simulink model "full_obs"  (Simulink 7.3)
settings: Solver=ode3  StartTime=0.0  StopTime=1500  FixedStep=1  RelTol=1e-3
settings Model: Creator=alkis  LastModifiedBy=alkis
settings DataIOCC: MaxDataPoints=10000  SaveState=on

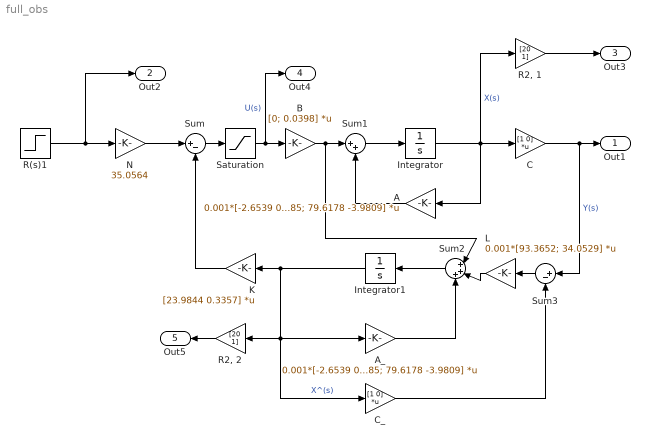
== system full_obs ==
  A : Gain  Gain=0.001*[-2.6539 0.0885; 79.6178 -3.9809]  Multiplication=Matrix(K*u)  ParameterDataType=fixdt(1, 16)  ParameterScaling=2^0  OutDataType=fixdt(1, 16)  OutScaling=2^0
  A_ : Gain  Gain=0.001*[-2.6539 0.0885; 79.6178 -3.9809]  Multiplication=Matrix(K*u)  ParameterDataType=fixdt(1, 16)  ParameterScaling=2^0  OutDataType=fixdt(1, 16)  OutScaling=2^0
  B : Gain  Gain=[0; 0.0398]  Multiplication=Matrix(K*u)  ParameterDataType=fixdt(1, 16)  ParameterScaling=2^0  OutDataType=fixdt(1, 16)  OutScaling=2^0
  C : Gain  Gain=[1 0]  Multiplication=Matrix(K*u)  ParameterDataType=fixdt(1, 16)  ParameterScaling=2^0  OutDataType=fixdt(1, 16)  OutScaling=2^0
  C_ : Gain  Gain=[1 0]  Multiplication=Matrix(K*u)  ParameterDataType=fixdt(1, 16)  ParameterScaling=2^0  OutDataType=fixdt(1, 16)  OutScaling=2^0
  Integrator : Integrator
  Integrator1 : Integrator
  K : Gain  Gain=[23.9844 0.3357]  Multiplication=Matrix(K*u)  ParameterDataType=fixdt(1, 16)  ParameterScaling=2^0  OutDataType=fixdt(1, 16)  OutScaling=2^0
  L : Gain  Gain=0.001*[93.3652; 34.0529]  Multiplication=Matrix(K*u)  ParameterDataType=fixdt(1, 16)  ParameterScaling=2^0  OutDataType=fixdt(1, 16)  OutScaling=2^0
  N : Gain  Gain=35.0564  ParameterDataType=fixdt(1, 16)  ParameterScaling=2^0  OutDataType=fixdt(1, 16)  OutScaling=2^0
  R(s)1 : Step  Time=0  After=0.1  SampleTime=0
  "R2, 1" : Gain  Gain=[20 1]  ParameterDataType=fixdt(1, 16)  ParameterScaling=2^0  OutDataType=fixdt(1, 16)  OutScaling=2^0
  "R2, 2" : Gain  Gain=[20 1]  ParameterDataType=fixdt(1, 16)  ParameterScaling=2^0  OutDataType=fixdt(1, 16)  OutScaling=2^0
  Saturation : Saturate  UpperLimit=3  LowerLimit=0  OutDataType=fixdt(1, 16)  OutScaling=2^0
  Sum : Sum  Inputs=|+-  OutDataType=fixdt(1, 16)  OutScaling=2^0
  Sum1 : Sum  Inputs=|++  OutDataType=fixdt(1, 16)  OutScaling=2^0
  Sum2 : Sum  Inputs=|+++  OutDataType=fixdt(1, 16)  OutScaling=2^0
  Sum3 : Sum  Inputs=|+-  OutDataType=fixdt(1, 16)  OutScaling=2^0
  Out1 : Outport  OutDataType=fixdt(1, 16)  OutScaling=2^0
  Out2 : Outport  Port=2  OutDataType=fixdt(1, 16)  OutScaling=2^0
  Out3 : Outport  Port=3  OutDataType=fixdt(1, 16)  OutScaling=2^0
  Out4 : Outport  Port=4  OutDataType=fixdt(1, 16)  OutScaling=2^0
  Out5 : Outport  Port=5  OutDataType=fixdt(1, 16)  OutScaling=2^0
  wires:
  N/1 -> Sum/1
  C/1 -> Out1/1, Sum3/1  "Y(s)"
  Integrator/1 -> C/1, "R2, 1"/1, A/1  "X(s)"
  Sum/1 -> Saturation/1
  K/1 -> Sum/2
  Saturation/1 -> Out4/1, B/1  "U(s)"
  A/1 -> Sum1/2
  Sum1/1 -> Integrator/1
  "R2, 1"/1 -> Out3/1
  Sum2/1 -> Integrator1/1
  A_/1 -> Sum2/3
  C_/1 -> Sum3/2
  Sum3/1 -> L/1
  L/1 -> Sum2/2
  B/1 -> Sum1/1, Sum2/1
  Integrator1/1 -> K/1, A_/1, C_/1, "R2, 2"/1  "X^(s)"
  "R2, 2"/1 -> Out5/1
  R(s)1/1 -> N/1, Out2/1
